simulink model "adjustablePIDcontrol"  (R2014b)
settings: Solver=FixedStepDiscrete  StartTime=0.0  StopTime=inf  FixedStep=1e-3  RelTol=1e-3
settings Model: Creator=wasonj  LastModifiedBy=Sean
settings DataIOCC: MaxDataPoints=10000  SignalLoggingSaveFormat=ModelDataLogs
settings OptimizationCC: ExpressionDepthLimit=2147483647
settings DebuggingCC: UnderspecifiedInitializationDetection=Classic  MergeDetectMultiDrivingBlocksExec=none  FcnCallInpInsideContextMsg=EnableAllAsWarning  StateNameClashWarn=warning
settings RTWCC: SystemTargetFile=catsdll.tlc  TemplateMakefile=catsdll_vc.tmf  Description=CATS DLL Real-Time Target  ProcessScript=catsdll_make_rtw_hook
settings STFCustomTargetCC: ModelReferenceCompliant=off  GeneratePreprocessorConditionals=Disable all  MATLABClassNameForMDSCustomization=Simulink.SoftwareTarget.TargetSpecificTriggerConfigurationBase  SystemTargetFile=catsdll.tlc

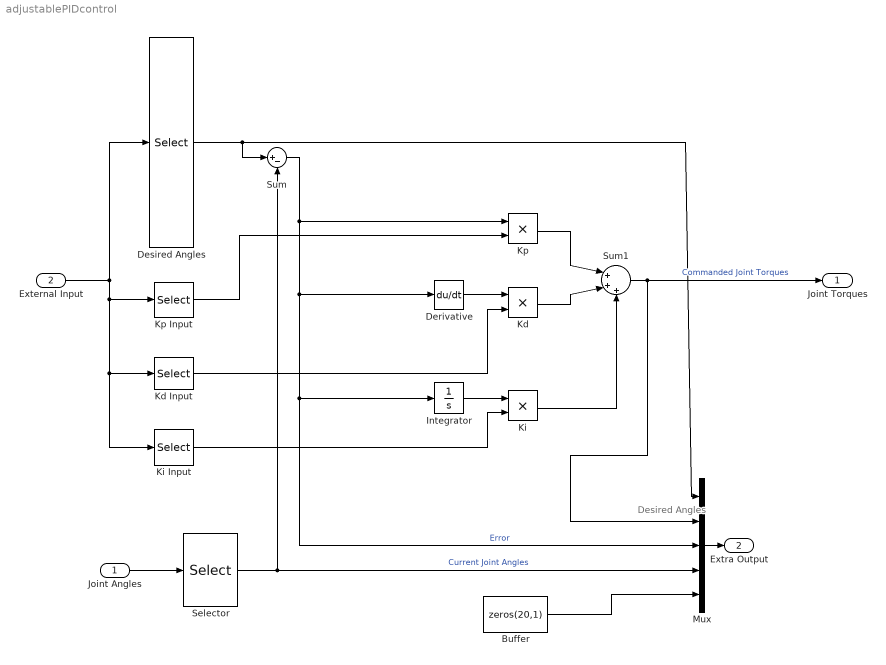
== system adjustablePIDcontrol ==
  note: Desired Angles
  Joint Angles : Inport  PortDimensions=6
  External Input : Inport  Port=2  PortDimensions=16
  Buffer : Constant  Value=zeros(20,1)
  Derivative : Derivative
  Desired Angles : Selector  InputPortWidth=16  Indices=[1:3]
  Integrator : Integrator  LimitOutput=on
  Kd : Product
  Kd Input : Selector  InputPortWidth=16  Indices=[7:9]
  Ki : Product
  Ki Input : Selector  InputPortWidth=16  Indices=[10:12]
  Kp : Product
  Kp Input : Selector  InputPortWidth=16  Indices=[4:6]
  Mux : Mux  Inputs=5
  Selector : Selector  InputPortWidth=6  Indices=1:3
  Sum : Sum  Inputs=|+-
  Sum1 : Sum  Inputs=|+++
  Joint Torques : Outport  PortDimensions=3
  Extra Output : Outport  Port=2  PortDimensions=32
  wires:
  Joint Angles/1 -> Selector/1
  Selector/1 -> Sum/2, Mux/4  "Current Joint Angles"
  Sum/1 -> Kp/1, Mux/3, Integrator/1, Derivative/1  "Error"
  Sum1/1 -> Joint Torques/1, Mux/2  "Commanded Joint Torques"
  Mux/1 -> Extra Output/1
  Buffer/1 -> Mux/5
  Desired Angles/1 -> Sum/1, Mux/1
  External Input/1 -> Kd Input/1, Ki Input/1, Kp Input/1, Desired Angles/1
  Kd/1 -> Sum1/2
  Ki/1 -> Sum1/3
  Kp/1 -> Sum1/1
  Kp Input/1 -> Kp/2
  Kd Input/1 -> Kd/2
  Derivative/1 -> Kd/1
  Integrator/1 -> Ki/1
  Ki Input/1 -> Ki/2
